simulink model "simulation_file"  (R2023b)
settings: Solver=VariableStepAuto  StartTime=0.0  StopTime=10.0  RelTol=1e-3
values from neighbouring files (symbols this model uses):
  m = sqrt(det(JJt))    [computeManipulabilityJacobian.m]
  maxWaypoints = 20    [createWaypointData.m]    (also in importfrankaEmikaPanda.m)
  ts = 0.01    [createWaypointData.m]    (also in importfrankaEmikaPanda.m; matlab_obstacle_avoidance.m = 0.001; matlab_obstacle_avoidance_for_code_gen.m = 0.001)
  waypointTimes = 0:4:16    [createWaypointData.m]    (also in importfrankaEmikaPanda.m; matlab_obstacle_avoidance.m; matlab_obstacle_avoidance_for_code_gen.m)
  X = X + v0(1)    [plotCylinder.m]    (also in plotSphere.m = X + center(1))
  Y = Y + v0(2)    [plotCylinder.m]    (also in plotSphere.m = Y + center(2))
  Z = Z + v0(3)    [plotCylinder.m]    (also in plotSphere.m = Z + center(3))
undefined symbols (not defined in the file or in its folder): diff
libraries: sm_lib x98, nesl_utility x15, robotmaniplib x13, robotcorelib x6, trajExampleUtils x6
(part 3 of 3)

== system simulation_file/Franka Emika Panda/Franka_Robot/panda_rightfinger ==
  Inertia : sm_lib/Body Elements/Inertia  InertiaType=Custom  Mass=0  MassUnits=kg  CenterOfMass=[0, 0, 0]  CenterOfMassUnits=m  MomentsOfInertia=[0, 0, 0]  MomentsOfInertiaUnits=kg*m^2  ProductsOfInertia=[0, 0, 0]  ProductsOfInertiaUnits=kg*m^2  GraphicType=None  MarkerShape=Inertia  MarkerSize=20  GraphicVisPropType=SimpleVisualProperties  GraphicDiffuseColor=[0.5 0.5 0.5]  GraphicSpecularColor=[0.5 0.5 0.5 1.0]  GraphicAmbientColor=[0.15 0.15 0.15 1.0]  GraphicEmissiveColor=[0.0 0.0 0.0 1.0]  GraphicShininess=75  GraphicOpacity=1.0
  InertiaOriginTransform : sm_lib/Frames and Transforms/Rigid Transform  TranslationMethod=Cartesian  TranslationStandardOffset=0  TranslationStandardOffsetUnits=m  TranslationStandardAxis=+Z  TranslationCartesianOffset=[0, 0, 0]  TranslationCartesianOffsetUnits=m  TranslationROffset=0  TranslationROffsetUnits=m  TranslationZOffset=0  TranslationZOffsetUnits=m  TranslationThetaOffset=0  TranslationThetaOffsetUnits=deg  RotationMethod=RotationSequence  RotationAngleUnits=deg  RotationStandardAxis=+Z  RotationAngle=0.0  RotationArbitraryAxis=[0 0 1]  FollAlignAxisA=+X  BaseAlignAxisA=+Y  FollAlignAxisB=+Y  BaseAlignAxisB=+Z  RotationSequenceAxes=BaseAxes  RotationSequence=XYZ  RotationSequenceAngles=[0, 0, 0]  RotationSequenceAnglesUnits=rad  RotationMatrix=[1 0 0; 0 1 0; 0 0 1]  Quaternion=[1 0 0 0]
  ReferenceFrame : sm_lib/Frames and Transforms/Reference Frame
  Visual : sm_lib/Body Elements/File Solid  ExtGeomFileName=/home/shobhit/Documents/MATLAB/SupportPackages/R2023b/toolbox/robotics/supportpackages/robotlibrary/Robots/franka_description/meshes/visual/finger.stl  UnitType=Custom  ExtGeomFileUnits=m  StepReaderType=HEX  ExportConvexHullGeometry=off  InertiaType=Custom  Mass=0  MassUnits=kg  CenterOfMass=[0, 0, 0]  CenterOfMassUnits=m  MomentsOfInertia=[0, 0, 0]  MomentsOfInertiaUnits=kg*m^2  ProductsOfInertia=[0, 0, 0]  ProductsOfInertiaUnits=kg*m^2  BasedOnType=DensityFromFile  Density=1000  DensityUnits=kg/m^3  DoExposeReferenceFrame=on  SerializedFrames=<Frames/>  GraphicType=FromGeometry  MarkerShape=Sphere  MarkerSize=10  GraphicVisPropType=SimpleVisualProperties  GraphicDiffuseColor=[0.5, 0.5, 0.5]  GraphicSpecularColor=[0.5 0.5 0.5 1.0]  GraphicAmbientColor=[0.15 0.15 0.15 1.0]  GraphicEmissiveColor=[0.0 0.0 0.0 1.0]  GraphicShininess=75  GraphicOpacity=1
  VisualOriginTransform : sm_lib/Frames and Transforms/Rigid Transform  TranslationMethod=Cartesian  TranslationStandardOffset=0  TranslationStandardOffsetUnits=m  TranslationStandardAxis=+Z  TranslationCartesianOffset=[0, 0, 0]  TranslationCartesianOffsetUnits=m  TranslationROffset=0  TranslationROffsetUnits=m  TranslationZOffset=0  TranslationZOffsetUnits=m  TranslationThetaOffset=0  TranslationThetaOffsetUnits=deg  RotationMethod=RotationSequence  RotationAngleUnits=deg  RotationStandardAxis=+Z  RotationAngle=0.0  RotationArbitraryAxis=[0 0 1]  FollAlignAxisA=+X  BaseAlignAxisA=+Y  FollAlignAxisB=+Y  BaseAlignAxisB=+Z  RotationSequenceAxes=BaseAxes  RotationSequence=XYZ  RotationSequenceAngles=[0, 0, -3.141592653589587]  RotationSequenceAnglesUnits=rad  RotationMatrix=[1 0 0; 0 1 0; 0 0 1]  Quaternion=[1 0 0 0]
  panda_finger_joint2_AxisInvTransform : sm_lib/Frames and Transforms/Rigid Transform  TranslationMethod=Cartesian  TranslationStandardOffset=0  TranslationStandardOffsetUnits=m  TranslationStandardAxis=+Z  TranslationCartesianOffset=[0, 0, 0]  TranslationCartesianOffsetUnits=m  TranslationROffset=0  TranslationROffsetUnits=m  TranslationZOffset=0  TranslationZOffsetUnits=m  TranslationThetaOffset=0  TranslationThetaOffsetUnits=deg  RotationMethod=ArbitraryAxis  RotationAngleUnits=rad  RotationStandardAxis=+Z  RotationAngle=1.570796326794897  RotationArbitraryAxis=[1, 0, 0]  FollAlignAxisA=+X  BaseAlignAxisA=+Y  FollAlignAxisB=+Y  BaseAlignAxisB=+Z  RotationSequenceAxes=FollowerAxes  RotationSequence=XYX  RotationSequenceAngles=[0 0 0]  RotationSequenceAnglesUnits=deg  RotationMatrix=[1 0 0; 0 1 0; 0 0 1]  Quaternion=[1 0 0 0]
  F : PMIOPort  Side=Left
  connections:
  Inertia/RConn1 -- InertiaOriginTransform/RConn1
  ReferenceFrame/RConn1 -- InertiaOriginTransform/LConn1 -- VisualOriginTransform/LConn1 -- panda_finger_joint2_AxisInvTransform/LConn1
  Visual/RConn1 -- VisualOriginTransform/RConn1
  panda_finger_joint2_AxisInvTransform/RConn1 -- F/RConn1

== system simulation_file/Trajectory Generation/Rotation Trajectory/Extract Trajectory Segment ==
  segIdx : Inport
  waypointTimes : Inport  Port=2
  orientations : Inport  Port=3
  Enable : EnablePort  PropagateVarSize=During execution
  MATLAB Function : MATLAB Function  TreatAsAtomicUnit=on
  q0 : Outport  VectorParamsAs1DForOutWhenUnconnected=off
  qf : Outport  Port=2  VectorParamsAs1DForOutWhenUnconnected=off
  timeInterval : Outport  Port=3  VectorParamsAs1DForOutWhenUnconnected=off
  wires:
  segIdx/1 -> MATLAB Function/1(segIdx)
  MATLAB Function/1(q0) -> q0/1
  MATLAB Function/3(timeInterval) -> timeInterval/1
  orientations/1 -> MATLAB Function/3(orientations)
  MATLAB Function/2(qf) -> qf/1
  waypointTimes/1 -> MATLAB Function/2(waypointTimes)

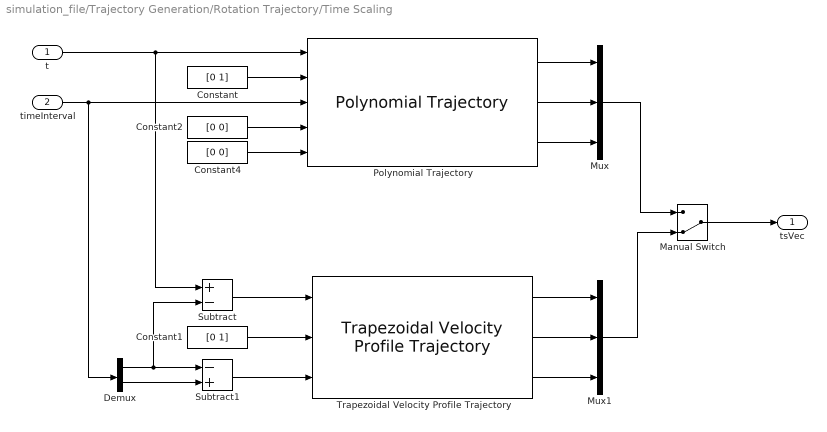
== system simulation_file/Trajectory Generation/Rotation Trajectory/Time Scaling ==
  t : Inport
  timeInterval : Inport  Port=2
  Constant : Constant  Value=[0 1]  VectorParams1D=off
  Constant1 : Constant  Value=[0 1]  VectorParams1D=off
  Constant2 : Constant  Value=[0 0]  VectorParams1D=off
  Constant4 : Constant  Value=[0 0]  VectorParams1D=off
  Demux : Demux  Outputs=2
  Manual Switch : ManualSwitch  CurrentSetting=0
  Mux : Mux  Inputs=3
  Mux1 : Mux  Inputs=3
  Polynomial Trajectory : robotcorelib/Polynomial Trajectory  WaypointSource=External  Waypoints=[ 0, 2, 1, 5, 0; -1, 3, 1, 4, 4 ]  TimePoints=[ 0, 1, 2, 3, 4 ]  TimeInterval=[ 1, 4 ]  Method=Quintic Polynomial  ParameterSource=External  VelocityBoundaryCondition=zeros( 2, 5 )  AccelerationBoundaryCondition=zeros( 2, 5 )  SimulateUsing=Interpreted execution
  Subtract : Sum  Inputs=+-
  Subtract1 : Sum  Inputs=-+
  Trapezoidal Velocity Profile Trajectory : robotcorelib/Trapezoidal Velocity Profile Trajectory  WaypointSource=External  Waypoints=[ 0, -0.5, -1; 0, 0.5, 1 ]  NumParams=1  Parameter1=End Time  Parameter2=End Time  ParameterSource=External  PeakVelocity=[ 2; 2 ]  Acceleration=[ 1; 2 ]  EndTime=[ 1; 1 ]  AccelTime=[ 1; 2 ]  SimulateUsing=Interpreted execution
  tsVec : Outport  VectorParamsAs1DForOutWhenUnconnected=off
  wires:
  Manual Switch/1 -> tsVec/1
  Polynomial Trajectory/3 -> Mux/3
  Polynomial Trajectory/1 -> Mux/1
  Constant/1 -> Polynomial Trajectory/2
  Constant4/1 -> Polynomial Trajectory/5
  Constant2/1 -> Polynomial Trajectory/4
  Polynomial Trajectory/2 -> Mux/2
  t/1 -> Polynomial Trajectory/1, Subtract/1
  Mux/1 -> Manual Switch/1
  Trapezoidal Velocity Profile Trajectory/1 -> Mux1/1
  Trapezoidal Velocity Profile Trajectory/2 -> Mux1/2
  Trapezoidal Velocity Profile Trajectory/3 -> Mux1/3
  Mux1/1 -> Manual Switch/2
  Constant1/1 -> Trapezoidal Velocity Profile Trajectory/2
  timeInterval/1 -> Demux/1, Polynomial Trajectory/3
  Subtract1/1 -> Trapezoidal Velocity Profile Trajectory/3
  Demux/1 -> Subtract/2, Subtract1/1
  Subtract/1 -> Trapezoidal Velocity Profile Trajectory/1
  Demux/2 -> Subtract1/2

== matlab function simulation_file/MATLAB Function ==
  data: T input; translation output
function translation = extractTranslation(T)
    % Extract the translation vector from the transformation matrix
    translation = T(1:3,4);
end

== matlab function simulation_file/Jacobimatrix_to_ith_link/MATLAB Function ==
  data: T01 input; Jacobimatrix output; T02 input; T03 input; T04 input; T05 input; T06 input; T07 input; T0tcp input; to_ith_link input
function Jacobimatrix = fcn(T01,T02,T03,T04,T05,T06,T07,T0tcp,to_ith_link)

%Array of transformation matrices 
T = {T01,T02,T03,T04,T05,T06,T07,T0tcp};

numJoints = 7; % Number of joints
J = zeros(6, numJoints); % Initialize Jacobian matrix with zeros
    if to_ith_link == 8 
        T_end_effector = T0tcp;
    else
    % Compute the transformation to the end-effector or to_ith_link
    T_end_effector = T07;
    end
    
    end_effector_position = T_end_effector(1:3, 4);

    for i = 1:to_ith_link-1
        % Get the transformation matrix from the base frame to the ith joint
        T_i = T{i};

        % Extract the z-axis of the ith joint in base frame coordinates
        z_i = T_i(1:3, 1:3) * [0; 0; 1];

        % Position of the ith joint in base frame coordinates
        d_i = T_i(1:3, 4);

        % Linear velocity contribution: cross product of z-axis with the vector from joint i to the end-effector
        Jv_i = cross(z_i, (end_effector_position - d_i));

        % Angular velocity contribution: simply the z-axis for revolute joints
        Jw_i = z_i;

        % Fill in the ith column of the Jacobian matrix for joint i
        J(1:3, i) = Jv_i; % Upper part for linear velocity
        J(4:6, i) = Jw_i; % Lower part for angular velocity
    end

    % Columns of Jacobian corresponding to joints beyond to_ith_link are already initialized to zero
    Jacobimatrix = J;
end

== matlab function simulation_file/MATLAB Function1 ==
  data: qd input; qe output; qc input
function qe = computequatError(qd, qc)
    % Ensure the quaternions are normalized
    qd = qd / norm(qd);
    qc = qc / norm(qc);

    % Compute the conjugate of the current orientation quaternion
    qc_conj = [qc(1), -qc(2), -qc(3), -qc(4)];
    
    % Compute the quaternion error
    qe = quatmultiply(qd, qc_conj);
end

== matlab function simulation_file/MATLAB Function2 ==
  data: T input; quat output
function quat = tmatrix2quat(T)

% Make sure the rotation matrix is 3x3
R = T(1:3, 1:3);

% Preallocate the quaternion
quat = zeros(1, 4);

% Calculate the trace of the matrix
tr = trace(R);

% Check the value of the trace
if tr > 0
    S = sqrt(tr + 1.0) * 2; % S=4*qw
    quat(1) = 0.25 * S;
    quat(2) = (R(3,2) - R(2,3)) / S;
    quat(3) = (R(1,3) - R(3,1)) / S;
    quat(4) = (R(2,1) - R(1,2)) / S;
elseif (R(1,1) > R(2,2)) && (R(1,1) > R(3,3))
    S = sqrt(1.0 + R(1,1) - R(2,2) - R(3,3)) * 2; % S=4*qx
    quat(1) = (R(3,2) - R(2,3)) / S;
    quat(2) = 0.25 * S;
    quat(3) = (R(1,2) + R(2,1)) / S;
    quat(4) = (R(1,3) + R(3,1)) / S;
elseif R(2,2) > R(3,3)
    S = sqrt(1.0 + R(2,2) - R(1,1) - R(3,3)) * 2; % S=4*qy
    quat(1) = (R(1,3) - R(3,1)) / S;
    quat(2) = (R(1,2) + R(2,1)) / S;
    quat(3) = 0.25 * S;
    quat(4) = (R(2,3) + R(3,2)) / S;
else
    S = sqrt(1.0 + R(3,3) - R(1,1) - R(2,2)) * 2; % S=4*qz
    quat(1) = (R(2,1) - R(1,2)) / S;
    quat(2) = (R(1,3) + R(3,1)) / S;
    quat(3) = (R(2,3) + R(3,2)) / S;
    quat(4) = 0.25 * S;
end

% Normalize the quaternion
quat = quat / norm(quat);
end

== matlab function simulation_file/MATLAB Function3 ==
  data: q_err input; omega output; delta_t input
function omega = quatErrorToAngVel(q_err, delta_t)
    % Extract the scalar and vector parts from the quaternion error
    w = q_err(1);
    vec = q_err(2:4);

    % Calculate the rotation angle from the quaternion scalar part
    theta = 2 * acos(w);

    % Calculate sin(theta/2)
    sin_half_theta = sin(theta / 2);

    % Prevent division by very small numbers by ensuring sin(theta/2) is not too small
    if sin_half_theta < eps
        % For very small angles, use the linear approximation: omega = 2 * vec / delta_t
        omega = (2 / delta_t) * vec;
    else
        % For larger angles, calculate the angular velocity using the full formula
        omega = (2 * acos(w) / delta_t) * (vec / sin_half_theta);
    end
end

== matlab function simulation_file/Trajectory Generation/Rotation Trajectory/Get Trajectory Index ==
  data: hasChanged output; t input; segIdx output; waypointTimes input size=[1 maxWaypoints]
function [hasChanged,segIdx] = getTrajIdx(t,waypointTimes)

% Initialize previous index
persistent prevIdx
if isempty(prevIdx)
    prevIdx = 0;
end

% Find the trajectory segment index
segIndices = find(t>=waypointTimes);

% Limit the index value to the number of times minus one
% (This addresses the final time case)
segIdx = min(segIndices(end),numel(waypointTimes)-1);

% Determine whether the index has changed from the previous time step
if prevIdx == segIdx
    hasChanged = false;
else
    hasChanged = true;
    prevIdx = segIdx;
end

end

== matlab function simulation_file/Trajectory Generation/Rotation Trajectory/Extract Trajectory Segment/MATLAB Function ==
  data: segIdx input; waypointTimes input size=[1 maxWaypoints]; q0 output size=[1 4]; orientations input size=[3 maxWaypoints]; qf output size=[1 4]; timeInterval output size=[1 2]
function [q0, qf, timeInterval] = createRotationTrajSegment(segIdx,waypointTimes,orientations)

% Extract the time interval, initial, and final quaternions for the segment
timeInterval = waypointTimes(segIdx:segIdx+1);
q0 = eul2quat(orientations(:,segIdx)');
qf = eul2quat(orientations(:,segIdx+1)');

end
